simulink model "AB_Final_of_MPC_Bandwidth_Result_UnbalancedNew"  (R2022b)
settings: Solver=FixedStepDiscrete  StartTime=0.0  StopTime=Inf  FixedStep=100e-6  RelTol=1e-3  EnableMultiTasking=on
undefined symbols (not defined in the file): C28x, CPU1, CPU2, CurrentBypassValue, DiscIntNeverNeededParam, Down, GPTRIP1SEL, TZ1, Up
libraries: c2802xlib x20, simulink x17, dspstat3 x13, eeGeneralControl x10, c2837xDlib x5, c280xlib x5, PID_Lib x4, c2000lib x1, spsAlphaBetaZerotoabcLib x1
(part 10 of 10)

== system AB_Final_of_MPC_Bandwidth_Result_UnbalancedNew/Subsystem1/GridCurrentSecondPrediction/CostFunctionofVoltageVectors/CostFunctionVoltage4/DGridCurrentSecondPrediction_Voltage4 ==
  MPCC_f32Predictionterm_A : Inport
  MPCC_f32Predictionterm_B : Inport  Port=2
  MPCC_f32Predictionterm_C : Inport  Port=3
  MPCC_f32DGridCurrent_K_1 : Inport  Port=4
  MPCC_f32QGridCurrent_K_1 : Inport  Port=5
  MPCC_f32DGridVoltage : Inport  Port=6
  MPCC_f32DVoltageVector4 : Inport  Port=7
  Add1 : Sum  Inputs=+++-
  Gain : Gain  Gain=0
  Product : Product
  Product1 : Product
  Product2 : Product  OutDataTypeStr=Inherit: Inherit via back propagation
  Product4 : Product
  MPCC_f32DGridCurrent_K_2_Voltage4 : Outport
  wires:
  [MPCC_f32DGridCurrent_K_1] -> Product/2
  MPCC_f32Predictionterm_A/1 -> [MPCC_f32Predictionterm_A]
  [MPCC_f32DGridVoltage] -> Product2/2
  Product1/1 -> Gain/1
  [MPCC_f32Predictionterm_C] -> Product1/1
  Product/1 -> Add1/1
  [MPCC_f32DVoltageVector4] -> Product4/2
  MPCC_f32DGridVoltage/1 -> [MPCC_f32DGridVoltage]
  [MPCC_f32Predictionterm_A] -> Product/1
  [MPCC_f32Predictionterm_B] -> Product4/1
  [MPCC_f32Predictionterm_B] -> Product2/1
  [MPCC_f32QGridCurrent_K_1] -> Product1/2
  MPCC_f32DGridCurrent_K_1/1 -> [MPCC_f32DGridCurrent_K_1]
  MPCC_f32QGridCurrent_K_1/1 -> [MPCC_f32QGridCurrent_K_1]
  MPCC_f32Predictionterm_C/1 -> [MPCC_f32Predictionterm_C]
  MPCC_f32Predictionterm_B/1 -> [MPCC_f32Predictionterm_B]
  Add1/1 -> MPCC_f32DGridCurrent_K_2_Voltage4/1
  MPCC_f32DVoltageVector4/1 -> [MPCC_f32DVoltageVector4]
  Product2/1 -> Add1/3
  Product4/1 -> Add1/4
  Gain/1 -> Add1/2

== system AB_Final_of_MPC_Bandwidth_Result_UnbalancedNew/Subsystem1/GridCurrentSecondPrediction/CostFunctionofVoltageVectors/CostFunctionVoltage4/QGridCurrentSecondPrediction_Voltage4 ==
  MPCC_f32Predictionterm_A : Inport
  MPCC_f32Predictionterm_B : Inport  Port=2
  MPCC_f32Predictionterm_C : Inport  Port=3
  MPCC_f32DGridCurrent_K_1 : Inport  Port=4
  MPCC_f32QGridCurrent_K_1 : Inport  Port=5
  MPCC_f32QGridVoltage : Inport  Port=6
  MPCC_f32QVoltageVector4 : Inport  Port=7
  Add1 : Sum  Inputs=+-+-
  Gain : Gain  Gain=0
  Product : Product
  Product1 : Product
  Product2 : Product  OutDataTypeStr=Inherit: Inherit via back propagation
  Product4 : Product  OutDataTypeStr=Inherit: Inherit via back propagation
  MPCC_f32QGridCurrent_K_2_Voltage4 : Outport
  wires:
  [MPCC_f32QGridCurrent_K_1] -> Product/2
  MPCC_f32Predictionterm_A/1 -> [MPCC_f32Predictionterm_A]
  [MPCC_f32QGridVoltage] -> Product2/2
  Product1/1 -> Gain/1
  [MPCC_f32Predictionterm_C] -> Product1/1
  Product/1 -> Add1/1
  [MPCC_f32QVoltageVector4] -> Product4/2
  [MPCC_f32Predictionterm_A] -> Product/1
  [MPCC_f32Predictionterm_B] -> Product4/1
  [MPCC_f32Predictionterm_B] -> Product2/1
  [MPCC_f32DGridCurrent_K_1] -> Product1/2
  MPCC_f32DGridCurrent_K_1/1 -> [MPCC_f32DGridCurrent_K_1]
  MPCC_f32QGridCurrent_K_1/1 -> [MPCC_f32QGridCurrent_K_1]
  MPCC_f32Predictionterm_C/1 -> [MPCC_f32Predictionterm_C]
  MPCC_f32QGridVoltage/1 -> [MPCC_f32QGridVoltage]
  MPCC_f32Predictionterm_B/1 -> [MPCC_f32Predictionterm_B]
  Add1/1 -> MPCC_f32QGridCurrent_K_2_Voltage4/1
  MPCC_f32QVoltageVector4/1 -> [MPCC_f32QVoltageVector4]
  Product2/1 -> Add1/3
  Product4/1 -> Add1/4
  Gain/1 -> Add1/2

== system AB_Final_of_MPC_Bandwidth_Result_UnbalancedNew/Subsystem1/GridCurrentSecondPrediction/CostFunctionofVoltageVectors/CostFunctionVoltage5/CostFunctionVoltage5 ==
  MPCC_f32DGridCurrentReference : Inport
  MPCC_f32QGridCurrentReference : Inport  Port=2
  MPCC_f32DGridCurrent_K_2_Voltage5 : Inport  Port=3
  MPCC_f32QGridCurrent_K_2_Voltage5 : Inport  Port=4
  MPCC_f32DGridCurrent : Inport  Port=5
  MPCC_f32QGridCurrent : Inport  Port=6
  MPCC_f32DGridCurrent1 : Inport  Port=7
  MPCC_f32QGridCurrent1 : Inport  Port=8
  Abs{,1..5} (6 alike) : Abs  SaturateOnIntegerOverflow=off
  Add{,2..6} (6 alike) : Sum  Inputs=+-
  Add1 : Sum  Inputs=++++++
  Constant : Constant  Value=single(0)
  Constant1 : Constant  Value=single(0)
  Gain : Gain
  Gain1 : Gain
  Gain2 : Gain  Gain=0
  Gain3 : Gain  Gain=0
  Square : Math  Operator=square
  Square1 : Math  Operator=square
  MPCC_f32CostFunction_Voltage5 : Outport
  wires:
  MPCC_f32QGridCurrentReference/1 -> [MPCC_f32QGridCurrentReference]
  MPCC_f32DGridCurrentReference/1 -> [MPCC_f32DGridCurrentReference]
  MPCC_f32QGridCurrent_K_2_Voltage5/1 -> [MPCC_f32QGridCurrent_K_2_Voltage5]
  MPCC_f32DGridCurrent_K_2_Voltage5/1 -> [MPCC_f32DGridCurrent_K_2_Voltage5]
  [MPCC_f32DGridCurrentReference] -> Add/1
  [MPCC_f32DGridCurrent_K_2_Voltage5] -> Add/2
  [MPCC_f32QGridCurrentReference] -> Add2/1
  [MPCC_f32QGridCurrent_K_2_Voltage5] -> Add2/2
  MPCC_f32QGridCurrent/1 -> [MPCC_f32QGridCurrent]
  MPCC_f32DGridCurrent/1 -> [MPCC_f32DGridCurrent]
  [MPCC_f32QGridCurrent] -> Add4/1
  Add4/1 -> Abs3/1
  Add3/1 -> Abs2/1
  [MPCC_f32QGridCurrent_K_2_Voltage5] -> Add4/2
  [MPCC_f32DGridCurrent] -> Add3/1
  [MPCC_f32DGridCurrent_K_2_Voltage5] -> Add3/2
  Abs2/1 -> Gain/1
  Abs3/1 -> Gain1/1
  Add1/1 -> MPCC_f32CostFunction_Voltage5/1
  Gain/1 -> Add1/3
  Gain1/1 -> Add1/4
  Abs1/1 -> Add1/2
  Add2/1 -> Abs1/1
  Abs/1 -> Add1/1
  Add/1 -> Abs/1
  MPCC_f32DGridCurrent1/1 -> [MPCC_f32DGridCurrent1]
  MPCC_f32QGridCurrent1/1 -> [MPCC_f32QGridCurrent1]
  Constant/1 -> Add5/1
  Add5/1 -> Abs4/1
  Add6/1 -> Abs5/1
  Abs4/1 -> Gain2/1
  Constant1/1 -> Add6/1
  [MPCC_f32DGridCurrent1] -> Add6/2
  [MPCC_f32QGridCurrent1] -> Add5/2
  Gain2/1 -> Add1/6
  Abs5/1 -> Gain3/1
  Gain3/1 -> Add1/5

== system AB_Final_of_MPC_Bandwidth_Result_UnbalancedNew/Subsystem1/GridCurrentSecondPrediction/CostFunctionofVoltageVectors/CostFunctionVoltage5/DGridCurrentSecondPrediction_Voltage5 ==
  MPCC_f32Predictionterm_A : Inport
  MPCC_f32Predictionterm_B : Inport  Port=2
  MPCC_f32Predictionterm_C : Inport  Port=3
  MPCC_f32DGridCurrent_K_1 : Inport  Port=4
  MPCC_f32QGridCurrent_K_1 : Inport  Port=5
  MPCC_f32DGridVoltage : Inport  Port=6
  MPCC_f32DVoltageVector5 : Inport  Port=7
  Add1 : Sum  Inputs=+++-
  Gain : Gain  Gain=0
  Product : Product
  Product1 : Product
  Product2 : Product  OutDataTypeStr=Inherit: Inherit via back propagation
  Product4 : Product
  MPCC_f32DGridCurrent_K_2_Voltage5 : Outport
  wires:
  [MPCC_f32DGridCurrent_K_1] -> Product/2
  MPCC_f32Predictionterm_A/1 -> [MPCC_f32Predictionterm_A]
  [MPCC_f32DGridVoltage] -> Product2/2
  Product1/1 -> Gain/1
  [MPCC_f32Predictionterm_C] -> Product1/1
  Product/1 -> Add1/1
  [MPCC_f32DVoltageVector5] -> Product4/2
  MPCC_f32DGridVoltage/1 -> [MPCC_f32DGridVoltage]
  [MPCC_f32Predictionterm_A] -> Product/1
  [MPCC_f32Predictionterm_B] -> Product4/1
  [MPCC_f32Predictionterm_B] -> Product2/1
  [MPCC_f32QGridCurrent_K_1] -> Product1/2
  MPCC_f32DGridCurrent_K_1/1 -> [MPCC_f32DGridCurrent_K_1]
  MPCC_f32QGridCurrent_K_1/1 -> [MPCC_f32QGridCurrent_K_1]
  MPCC_f32Predictionterm_C/1 -> [MPCC_f32Predictionterm_C]
  MPCC_f32Predictionterm_B/1 -> [MPCC_f32Predictionterm_B]
  Add1/1 -> MPCC_f32DGridCurrent_K_2_Voltage5/1
  MPCC_f32DVoltageVector5/1 -> [MPCC_f32DVoltageVector5]
  Product2/1 -> Add1/3
  Product4/1 -> Add1/4
  Gain/1 -> Add1/2

== system AB_Final_of_MPC_Bandwidth_Result_UnbalancedNew/Subsystem1/GridCurrentSecondPrediction/CostFunctionofVoltageVectors/CostFunctionVoltage5/QGridCurrentSecondPrediction_Voltage5 ==
  MPCC_f32Predictionterm_A : Inport
  MPCC_f32Predictionterm_B : Inport  Port=2
  MPCC_f32Predictionterm_C : Inport  Port=3
  MPCC_f32DGridCurrent_K_1 : Inport  Port=4
  MPCC_f32QGridCurrent_K_1 : Inport  Port=5
  MPCC_f32QGridVoltage : Inport  Port=6
  MPCC_f32QVoltageVector5 : Inport  Port=7
  Add1 : Sum  Inputs=+-+-
  Gain : Gain  Gain=0
  Product : Product
  Product1 : Product
  Product2 : Product  OutDataTypeStr=Inherit: Inherit via back propagation
  Product4 : Product
  MPCC_f32QGridCurrent_K_2_Voltage5 : Outport
  wires:
  [MPCC_f32QGridCurrent_K_1] -> Product/2
  MPCC_f32Predictionterm_A/1 -> [MPCC_f32Predictionterm_A]
  [MPCC_f32QGridVoltage] -> Product2/2
  Product1/1 -> Gain/1
  [MPCC_f32Predictionterm_C] -> Product1/1
  Product/1 -> Add1/1
  [MPCC_f32QVoltageVector5] -> Product4/2
  [MPCC_f32Predictionterm_A] -> Product/1
  [MPCC_f32Predictionterm_B] -> Product4/1
  [MPCC_f32Predictionterm_B] -> Product2/1
  [MPCC_f32DGridCurrent_K_1] -> Product1/2
  MPCC_f32DGridCurrent_K_1/1 -> [MPCC_f32DGridCurrent_K_1]
  MPCC_f32QGridCurrent_K_1/1 -> [MPCC_f32QGridCurrent_K_1]
  MPCC_f32Predictionterm_C/1 -> [MPCC_f32Predictionterm_C]
  MPCC_f32QGridVoltage/1 -> [MPCC_f32QGridVoltage]
  MPCC_f32Predictionterm_B/1 -> [MPCC_f32Predictionterm_B]
  Add1/1 -> MPCC_f32QGridCurrent_K_2_Voltage5/1
  MPCC_f32QVoltageVector5/1 -> [MPCC_f32QVoltageVector5]
  Product2/1 -> Add1/3
  Product4/1 -> Add1/4
  Gain/1 -> Add1/2

== system AB_Final_of_MPC_Bandwidth_Result_UnbalancedNew/Subsystem1/GridCurrentSecondPrediction/CostFunctionofVoltageVectors/CostFunctionVoltage6/CostFunctionVoltage6 ==
  MPCC_f32DGridCurrentReference : Inport
  MPCC_f32QGridCurrentReference : Inport  Port=2
  MPCC_f32DGridCurrent_K_2_Voltage6 : Inport  Port=3
  MPCC_f32QGridCurrent_K_2_Voltage6 : Inport  Port=4
  MPCC_f32DGridCurrent : Inport  Port=5
  MPCC_f32QGridCurrent : Inport  Port=6
  MPCC_f32DGridCurrent1 : Inport  Port=7
  MPCC_f32QGridCurrent1 : Inport  Port=8
  Abs{,1..5} (6 alike) : Abs  SaturateOnIntegerOverflow=off
  Add{,2..6} (6 alike) : Sum  Inputs=+-
  Add1 : Sum  Inputs=++++++
  Constant : Constant  Value=single(0)
  Constant1 : Constant  Value=single(0)
  Gain : Gain
  Gain1 : Gain
  Gain2 : Gain  Gain=0
  Gain3 : Gain  Gain=0
  Square : Math  Operator=square
  Square1 : Math  Operator=square
  MPCC_f32CostFunction_Voltage6 : Outport
  wires:
  MPCC_f32QGridCurrentReference/1 -> [MPCC_f32QGridCurrentReference]
  MPCC_f32DGridCurrentReference/1 -> [MPCC_f32DGridCurrentReference]
  MPCC_f32QGridCurrent_K_2_Voltage6/1 -> [MPCC_f32QGridCurrent_K_2_Voltage6]
  MPCC_f32DGridCurrent_K_2_Voltage6/1 -> [MPCC_f32DGridCurrent_K_2_Voltage6]
  [MPCC_f32DGridCurrentReference] -> Add/1
  [MPCC_f32DGridCurrent_K_2_Voltage6] -> Add/2
  [MPCC_f32QGridCurrentReference] -> Add2/1
  [MPCC_f32QGridCurrent_K_2_Voltage6] -> Add2/2
  MPCC_f32QGridCurrent/1 -> [MPCC_f32QGridCurrent]
  MPCC_f32DGridCurrent/1 -> [MPCC_f32DGridCurrent]
  [MPCC_f32QGridCurrent] -> Add4/1
  Add4/1 -> Abs3/1
  Add3/1 -> Abs2/1
  [MPCC_f32QGridCurrent_K_2_Voltage6] -> Add4/2
  [MPCC_f32DGridCurrent] -> Add3/1
  [MPCC_f32DGridCurrent_K_2_Voltage6] -> Add3/2
  Abs2/1 -> Gain/1
  Abs3/1 -> Gain1/1
  Add1/1 -> MPCC_f32CostFunction_Voltage6/1
  Gain/1 -> Add1/3
  Gain1/1 -> Add1/4
  Abs1/1 -> Add1/2
  Add2/1 -> Abs1/1
  Abs/1 -> Add1/1
  Add/1 -> Abs/1
  MPCC_f32DGridCurrent1/1 -> [MPCC_f32DGridCurrent1]
  MPCC_f32QGridCurrent1/1 -> [MPCC_f32QGridCurrent1]
  Constant/1 -> Add5/1
  Add5/1 -> Abs4/1
  Add6/1 -> Abs5/1
  Abs4/1 -> Gain2/1
  Constant1/1 -> Add6/1
  [MPCC_f32DGridCurrent1] -> Add6/2
  [MPCC_f32QGridCurrent1] -> Add5/2
  Gain2/1 -> Add1/6
  Abs5/1 -> Gain3/1
  Gain3/1 -> Add1/5

== system AB_Final_of_MPC_Bandwidth_Result_UnbalancedNew/Subsystem1/GridCurrentSecondPrediction/CostFunctionofVoltageVectors/CostFunctionVoltage6/DGridCurrentSecondPrediction_Voltage6 ==
  MPCC_f32Predictionterm_A : Inport
  MPCC_f32Predictionterm_B : Inport  Port=2
  MPCC_f32Predictionterm_C : Inport  Port=3
  MPCC_f32DGridCurrent_K_1 : Inport  Port=4
  MPCC_f32QGridCurrent_K_1 : Inport  Port=5
  MPCC_f32DGridVoltage : Inport  Port=6
  MPCC_f32DVoltageVector6 : Inport  Port=7
  Add1 : Sum  Inputs=+++-
  Gain : Gain  Gain=0
  Product : Product
  Product1 : Product
  Product2 : Product  OutDataTypeStr=Inherit: Inherit via back propagation
  Product4 : Product
  MPCC_f32DGridCurrent_K_2_Voltage6 : Outport
  wires:
  [MPCC_f32DGridCurrent_K_1] -> Product/2
  MPCC_f32Predictionterm_A/1 -> [MPCC_f32Predictionterm_A]
  [MPCC_f32DGridVoltage] -> Product2/2
  Product1/1 -> Gain/1
  [MPCC_f32Predictionterm_C] -> Product1/1
  Product/1 -> Add1/1
  [MPCC_f32DVoltageVector6] -> Product4/2
  MPCC_f32DGridVoltage/1 -> [MPCC_f32DGridVoltage]
  [MPCC_f32Predictionterm_A] -> Product/1
  [MPCC_f32Predictionterm_B] -> Product4/1
  [MPCC_f32Predictionterm_B] -> Product2/1
  [MPCC_f32QGridCurrent_K_1] -> Product1/2
  MPCC_f32DGridCurrent_K_1/1 -> [MPCC_f32DGridCurrent_K_1]
  MPCC_f32QGridCurrent_K_1/1 -> [MPCC_f32QGridCurrent_K_1]
  MPCC_f32Predictionterm_C/1 -> [MPCC_f32Predictionterm_C]
  MPCC_f32Predictionterm_B/1 -> [MPCC_f32Predictionterm_B]
  Add1/1 -> MPCC_f32DGridCurrent_K_2_Voltage6/1
  MPCC_f32DVoltageVector6/1 -> [MPCC_f32DVoltageVector6]
  Product2/1 -> Add1/3
  Product4/1 -> Add1/4
  Gain/1 -> Add1/2

== system AB_Final_of_MPC_Bandwidth_Result_UnbalancedNew/Subsystem1/GridCurrentSecondPrediction/CostFunctionofVoltageVectors/CostFunctionVoltage6/QGridCurrentSecondPrediction_Voltage6 ==
  MPCC_f32Predictionterm_A : Inport
  MPCC_f32Predictionterm_B : Inport  Port=2
  MPCC_f32Predictionterm_C : Inport  Port=3
  MPCC_f32DGridCurrent_K_1 : Inport  Port=4
  MPCC_f32QGridCurrent_K_1 : Inport  Port=5
  MPCC_f32QGridVoltage : Inport  Port=6
  MPCC_f32QVoltageVector6 : Inport  Port=7
  Add1 : Sum  Inputs=+-+-
  Gain : Gain  Gain=0
  Product : Product
  Product1 : Product
  Product2 : Product  OutDataTypeStr=Inherit: Inherit via back propagation
  Product4 : Product
  MPCC_f32QGridCurrent_K_2_Voltage6 : Outport
  wires:
  [MPCC_f32QGridCurrent_K_1] -> Product/2
  MPCC_f32Predictionterm_A/1 -> [MPCC_f32Predictionterm_A]
  [MPCC_f32QGridVoltage] -> Product2/2
  Product1/1 -> Gain/1
  [MPCC_f32Predictionterm_C] -> Product1/1
  Product/1 -> Add1/1
  [MPCC_f32QVoltageVector6] -> Product4/2
  [MPCC_f32Predictionterm_A] -> Product/1
  [MPCC_f32Predictionterm_B] -> Product4/1
  [MPCC_f32Predictionterm_B] -> Product2/1
  [MPCC_f32DGridCurrent_K_1] -> Product1/2
  MPCC_f32DGridCurrent_K_1/1 -> [MPCC_f32DGridCurrent_K_1]
  MPCC_f32QGridCurrent_K_1/1 -> [MPCC_f32QGridCurrent_K_1]
  MPCC_f32Predictionterm_C/1 -> [MPCC_f32Predictionterm_C]
  MPCC_f32QGridVoltage/1 -> [MPCC_f32QGridVoltage]
  MPCC_f32Predictionterm_B/1 -> [MPCC_f32Predictionterm_B]
  Add1/1 -> MPCC_f32QGridCurrent_K_2_Voltage6/1
  MPCC_f32QVoltageVector6/1 -> [MPCC_f32QVoltageVector6]
  Product2/1 -> Add1/3
  Product4/1 -> Add1/4
  Gain/1 -> Add1/2

== stateflow chart AB_Final_of_MPC_Bandwidth_Result_UnbalancedNew/Chart1 ==
  state GPin_FC [parallel]
    settings: executionOrder=1
    state Rate_100us
      on every(1,tic): send(GPin_FC);
    (default) -> GPin_FC.Rate_100us : /{send(GPin_FC);}
  state ADC_FC [parallel]
    settings: executionOrder=2
    state Rate_100us
      on every(1,tic): send(ADC_FC);
    (default) -> ADC_FC.Rate_100us : /{send(ADC_FC);}
  state PLL_FC [parallel]
    settings: executionOrder=3
    state Rate_100us
      on every(1,tic): send(PLL_FC);
    (default) -> PLL_FC.Rate_100us : /{send(PLL_FC);}
  state CurrentLoop_FC [parallel]
    settings: executionOrder=4
    state Rate_100us
      on every(1,tic): send(CurrentLoop_FC);
    (default) -> CurrentLoop_FC.Rate_100us : /{send(CurrentLoop_FC);}
  state VoltageLoop_FC [parallel]
    settings: executionOrder=5
    state Rate_1000us
      on every(10,tic): send(VoltageLoop_FC);
    (default) -> Rate_1000us : /{send(VoltageLoop_FC);}
  state GPout_FC [parallel]
    settings: executionOrder=6
    state Rate_100us
      on every(1,tic): send(GPout_FC);
    (default) -> GPout_FC.Rate_100us : /{send(GPout_FC);}
  events: ADC_FC output FUNCTION_CALL_EVENT; PLL_FC output FUNCTION_CALL_EVENT; tic input FUNCTION_CALL_EVENT; CurrentLoop_FC output FUNCTION_CALL_EVENT; VoltageLoop_FC output FUNCTION_CALL_EVENT; GPin_FC output FUNCTION_CALL_EVENT; GPout_FC output FUNCTION_CALL_EVENT

== matlab function AB_Final_of_MPC_Bandwidth_Result_UnbalancedNew/Subsystem1/MATLAB Function1 ==
  data: e_alpha input; alpha output; e_alpha_prime input; v_alpha input; v_alpha_prime input; e_beta input; e_beta_prime input; v_beta input; v_beta_prime input; Pref input; beta output
function [alpha,beta] = compute_vector(e_alpha, e_alpha_prime, v_alpha, v_alpha_prime, e_beta, e_beta_prime, v_beta, v_beta_prime,Pref)

DIOPC = (e_alpha^2 + e_alpha_prime^2)*(v_beta^2 + v_beta_prime^2) ...
      + (e_beta^2 + e_beta_prime^2)*(v_alpha^2 + v_alpha_prime^2) ...
      + 2*(v_alpha*v_beta_prime - v_alpha_prime*v_beta) ...
        *(e_alpha*e_beta_prime - e_alpha_prime*e_beta) ...
      - 2*(e_alpha*e_beta + e_alpha_prime*e_beta_prime) ...
        *(v_alpha*v_beta + v_alpha_prime*v_beta_prime);



row_1 = (e_beta_prime * v_beta_prime - e_beta * v_beta) * v_alpha ...
          - (e_beta * v_beta_prime + e_beta_prime * v_beta) * v_alpha_prime ...
          + (v_beta^2 + v_beta_prime^2) * e_alpha;

row_2 = (e_alpha_prime * v_alpha_prime - e_alpha * v_alpha) * v_beta ...
          - (e_alpha * v_alpha_prime + e_alpha_prime * v_alpha) * v_beta_prime ...
          + (v_alpha^2 + v_alpha_prime^2) * e_beta;

Gain = (4/3)*(Pref/DIOPC);

alpha=row_1*Gain;
beta=row_2*Gain;
end


% A0 = ((Valphap*Vbetan)-(Vbetap*Valphan));
% A1 = (Ealphap^(2)+Ealphan^(2)+Ebetap^(2)+Ebetan^(2));
% A2=  ((Ealphap*Ebetan)-(Ealphan*Ebetap));
% A3 = (Valphap^(2)+Valphan^(2)+Vbetap^(2)+Vbetan^(2));
% 
% denm = (A0*A1)+(A2*A3);
% 
% A4_ = (Valphap*Vbetan)-(Vbetap*Valphan);
% A4  = A4_*Ealphap;
% 
% A5_ = (Valphap*Vbetap)+(Vbetan*Valphan);
% A5  = A5_*Ealphan;
% 
% A6_ = (Vbetap^(2)+Vbetan^(2));
% A6  = A6_*Ebetan;
% 
% %%%%%%%%%%%
% 
% A7_ = (Valphap*Vbetan)-(Vbetap*Valphan);
% A7  = A7_*Ebetap;
% 
% A8_ = (Valphap*Vbetap)+(Vbetan*Valphan);
% A8  = -1*A8_*Ebetan;
% 
% A9_ = (Valphap^(2)+Vbetap^(2));
% A9  = -1*A9_*Ealphan;

% D= (Ealphap*Ebetan)-(Ealphan*Ebetap);
% 
% alpha= (Pref*Ebetan)/(D);
% beta= (-1*Pref*Ealphan)/(D);



% alpha = (2/3)*(A4+A5+A6)*(Pref/denm);
% beta = (2/3)*(A7+A8+A9)*(Pref/denm);

% 
% k1 = Ealphap*(Valphap^(2)+Vbetap^(2)) + Ealphan*((Vbetap*Vbetan)-(Valphap*Valphan)) - Ebetan*((Valphap*Vbetan)+(Vbetap*Valphan));
% 
% k2 = Ebetap*(Valphap^(2)+Vbetap^(2)) - Ealphan*((Valphap*Vbetan)+(Vbetap*Valphan)) + Ebetan*((Valphap*Valphan)-(Vbetap*Vbetan));
% 
% k3 = -1*Ealphan*(Valphan^(2)+Vbetan^(2)) + Ealphap*((Valphap*Valphan)-(Vbetap*Vbetan)) + Ebetap*((Valphap*Vbetan)+(Vbetap*Valphan));
% 
% k4 = -1*Ebetan*(Valphan^(2)+Vbetan^(2)) + Ealphap*((Valphap*Vbetan)+(Vbetap*Valphan)) + Ebetap*((Vbetap*Vbetan)-(Valphap*Valphan));
% 
% den= (k1*Ealphap) + (k2*Ebetap) + (k3*Ealphan) + (k4*Ebetan);
% 
% if den == 0
%     den = single(1000);
% end
% % 
% DOPC_Gain = (2/3)*(Pref/den);


% alpha= (k3-k1)*DOPC_Gain;
% beta = (k4-k2)*DOPC_Gain;
 
% Idp= -k1*DOPC_Gain;
% Iqp= -k2*DOPC_Gain;
% Idn= k3*DOPC_Gain;
% Iqn= k4*DOPC_Gain;

== matlab function AB_Final_of_MPC_Bandwidth_Result_UnbalancedNew/Subsystem1/MATLAB Function2 ==
  data: Ealpha input; alpha output; Ealpha_ input; Ebeta input; Ebeta_ input; Pref input; omega input; Ialpha input; beta output; Ibeta input
function [alpha,beta] = fcn(Ealpha,Ealpha_,Ebeta,Ebeta_,Pref,omega,Ialpha,Ibeta)

% v_alpha= Ealpha - (omega*20e-3*Ialpha);
% v_beta= Ebeta - (omega*20e-3*Ibeta);
% 
% 
% 
% v_alpha_= Ealpha_ - (omega*20e-3*Ialpha);
% v_beta_= Ebeta_ - (omega*20e-3*Ibeta);

% D = (Ebeta^2 + Ebeta_^2)*v_alpha^2 ...
%     + (2*v_beta_*Ebeta_*Ealpha ...
%     - 2*Ebeta_*Ealpha_*v_beta ...
%     - 2*Ebeta*Ealpha*v_beta ...
%     - 2*v_beta_*Ealpha_*Ebeta)*v_alpha ...
%     - 2*Ealpha*Ebeta_*v_alpha_*v_beta ...
%     + Ebeta^2*Ealpha_^2 ...
%     + Ealpha^2*v_beta^2 ...
%     - 2*Ealpha_*v_beta_*Ebeta*v_alpha_* ...
%     + Ebeta^2*v_beta_^2 ...
%     - 2*Ealpha*v_beta_*Ebeta*v_alpha_* ...
%     + 2*Ealpha_*Ebeta*v_alpha_*v_beta ...
%     + Ebeta_^2*v_alpha_^2 ...
%     + Ealpha_^2*v_beta^2 ...
%     + Ealpha_^2*v_beta_^2;
% 
% 
% prealpha = (Ebeta_*v_beta_ - Ebeta*v_beta)*v_alpha ...
%            - Ebeta_*v_alpha_*v_beta ...
%            - Ebeta*v_alpha_*v_beta_ ...
%            + Ealpha*v_beta^2 ...
%            + Ealpha*v_beta_^2;
% 
% prebeta  = (Ealpha_*v_beta_ + Ealpha*v_beta)*v_alpha ...
%            - Ealpha_*v_alpha_*v_beta ...
%            + Ealpha*v_alpha_*v_beta_ ...
%            - Ebeta*v_alpha_^2 ...
%            - Ebeta*v_alpha^2;

% Gain = (4/3)*(Pref/D);

alpha = ((2/3)*Pref*Ebeta_)/((Ealpha*Ebeta_)-(Ealpha_*Ebeta));
beta  = ((2/3)*-1*Pref*Ealpha_)/((Ealpha*Ebeta_)-(Ealpha_*Ebeta));


end

% A0 = ((Valphap*Vbetan)-(Vbetap*Valphan));
% A1 = (Ealphap^(2)+Ealphan^(2)+Ebetap^(2)+Ebetan^(2));
% A2=  ((Ealphap*Ebetan)-(Ealphan*Ebetap));
% A3 = (Valphap^(2)+Valphan^(2)+Vbetap^(2)+Vbetan^(2));
% 
% denm = (A0*A1)+(A2*A3);
% 
% A4_ = (Valphap*Vbetan)-(Vbetap*Valphan);
% A4  = A4_*Ealphap;
% 
% A5_ = (Valphap*Vbetap)+(Vbetan*Valphan);
% A5  = A5_*Ealphan;
% 
% A6_ = (Vbetap^(2)+Vbetan^(2));
% A6  = A6_*Ebetan;
% 
% %%%%%%%%%%%
% 
% A7_ = (Valphap*Vbetan)-(Vbetap*Valphan);
% A7  = A7_*Ebetap;
% 
% A8_ = (Valphap*Vbetap)+(Vbetan*Valphan);
% A8  = -1*A8_*Ebetan;
% 
% A9_ = (Valphap^(2)+Vbetap^(2));
% A9  = -1*A9_*Ealphan;

% D= (Ealphap*Ebetan)-(Ealphan*Ebetap);
% 
% alpha= (Pref*Ebetan)/(D);
% beta= (-1*Pref*Ealphan)/(D);



% alpha = (2/3)*(A4+A5+A6)*(Pref/denm);
% beta = (2/3)*(A7+A8+A9)*(Pref/denm);

% 
% k1 = Ealphap*(Valphap^(2)+Vbetap^(2)) + Ealphan*((Vbetap*Vbetan)-(Valphap*Valphan)) - Ebetan*((Valphap*Vbetan)+(Vbetap*Valphan));
% 
% k2 = Ebetap*(Valphap^(2)+Vbetap^(2)) - Ealphan*((Valphap*Vbetan)+(Vbetap*Valphan)) + Ebetan*((Valphap*Valphan)-(Vbetap*Vbetan));
% 
% k3 = -1*Ealphan*(Valphan^(2)+Vbetan^(2)) + Ealphap*((Valphap*Valphan)-(Vbetap*Vbetan)) + Ebetap*((Valphap*Vbetan)+(Vbetap*Valphan));
% 
% k4 = -1*Ebetan*(Valphan^(2)+Vbetan^(2)) + Ealphap*((Valphap*Vbetan)+(Vbetap*Valphan)) + Ebetap*((Vbetap*Vbetan)-(Valphap*Valphan));
% 
% den= (k1*Ealphap) + (k2*Ebetap) + (k3*Ealphan) + (k4*Ebetan);
% 
% if den == 0
%     den = single(1000);
% end
% % 
% DOPC_Gain = (2/3)*(Pref/den);


% alpha= (k3-k1)*DOPC_Gain;
% beta = (k4-k2)*DOPC_Gain;
 
% Idp= -k1*DOPC_Gain;
% Iqp= -k2*DOPC_Gain;
% Idn= k3*DOPC_Gain;
% Iqn= k4*DOPC_Gain;

== matlab function AB_Final_of_MPC_Bandwidth_Result_UnbalancedNew/Subsystem1/MATLAB Function3 ==
  data: ea input; alpha output; eb input; ea_p input; eb_p input; Pref input; beta output; omega input; ia input; ib input; ia1 input; ib1 input
function [alpha,beta] = fcn(ea,eb,ea_p,eb_p,Pref,omega,ia,ib,ia1,ib1)


% % 
% va = (ea) + (omega*18.5825e-3*ia1*1) - (ia1*0.55);
% vb = (eb) + (omega*18.5825e-3*ib1*1) - (ib1*0.55);
% va_p = (ea_p) - (omega*18.5825e-3*ia*1) - (ia*0.55);
% vb_p = (eb_p) - (omega*18.5825e-3*ib*1) - (ib*0.55);
% % 
% 
% 
% t1 = (va*vb_p - vb*va_p)*ea;
% t2 = (va*vb + vb_p*va_p)*ea_p;
% t3 = (vb*vb + vb_p*vb_p)*eb_p;
% 
% t4 = (va*vb_p - vb*va_p)*eb;
% t5 = (va*vb + vb_p*va_p)*eb_p;
% t6 = (va*va + va_p*va_p)*ea_p;
% 
% 
% prealpha = t1+t2+t3;
% prebeta  = t4-t5-t6;
% 
% delta = (va * vb_p - vb * va_p) * (ea^2 + ea_p^2 + eb^2 + eb_p^2) + ...
%         (ea * eb_p - ea_p * eb) * (va^2 + va_p^2 + vb^2 + vb_p^2);
% 
% gaint = (4/3)*(Pref/delta);
% 
% alpha = gaint*prealpha;
% beta  = gaint*prebeta;


% 
va = (ea) + (omega*9.5e-3*ia1*0.5) - (ia1*0.55*0);
vb = (eb) + (omega*9.5e-3*ib1*0.5) - (ib1*0.55*0);
va_p = (ea_p) - (omega*9.5e-3*ia*0.5) - (ia*0.55*0);
vb_p = (eb_p) - (omega*9.5e-3*ib*0.5) - (ib*0.55*0);
% 

term1 = (ea^2 + ea_p^2) * (vb^2 + vb_p^2);
term2 = (eb^2 + eb_p^2) * (va^2 + va_p^2);
term3 = 2 * (va * vb_p - va_p * vb) * (ea * eb_p - ea_p * eb);
term4 = 2 * (ea * eb + ea_p * eb_p) * (va * vb + va_p * vb_p);
% Combine the terms to find the final D_IOPC value
D_IOPC = (term1 + term2 + term3 - term4);


% delta = (va * vb_p - vb * va_p) * (ea^2 + ea_p^2 + eb^2 + eb_p^2) + ...
%         (ea * eb_p - ea_p * eb) * (va^2 + va_p^2 + vb^2 + vb_p^2);

Gain = (4/3)*(Pref/D_IOPC);

prealpha = ((eb_p * vb_p - eb * vb) * va) - ((eb * vb_p + eb_p * vb) * va_p) + ((vb^2 + vb_p^2) * ea);
prebeta  = ((ea_p * va_p - ea * va) * vb) - ((ea * va_p + ea_p * va) * vb_p) + ((va^2 + va_p^2) * eb);

alpha = Gain*prealpha;
beta =  Gain*prebeta;

% DIPC = (eb*ea_p - ea*eb_p);
% Gain = (Pref/DIPC)*(2/3);
% 
% alpha = Gain * -1 * eb_p;
% beta  = Gain * 1 * ea_p;

end
